simulink library "NullConstraintsBus"  (R2018b)
settings: Solver=VariableStepAuto  StartTime=0.0  StopTime=10.0  RelTol=1e-3
settings Model: Creator=RA24876  LastModifiedBy=RA24876
settings SFSimCC: SimUseLocalCustomCode=off
settings RTWCC: RTWUseLocalCustomCode=off
settings CodeAppCC: StateflowObjectComments=on

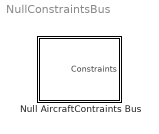
== system NullConstraintsBus ==
  Null AircraftContraints Bus : Subsystem  mask(Null AircraftConstraints Bus){}
      mask help: Creates an AircraftConstraints bus signal with all null values. Assign values to elements with a Bus Assignment block.

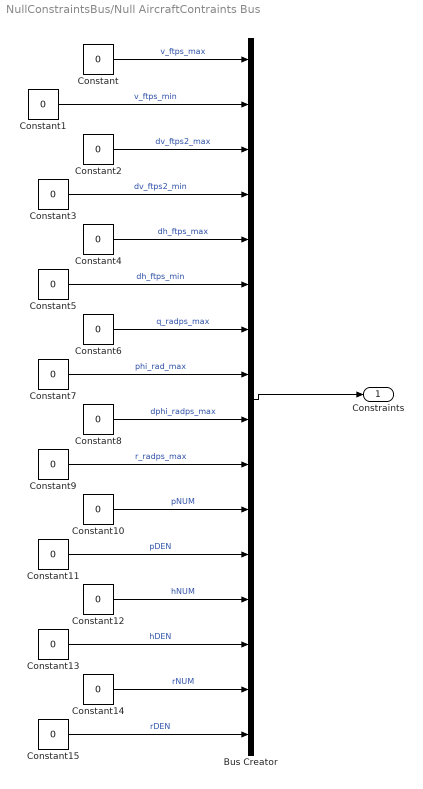
== system NullConstraintsBus/Null AircraftContraints Bus ==
  Bus Creator : BusCreator  Inputs=16  OutDataTypeStr=Bus: AircraftConstraints
      settings: InheritFromInputs=off
  Constant{,1..15} (16 alike) : Constant  Value=0
  Constraints : Outport  OutDataTypeStr=Bus: AircraftConstraints
  wires:
  Bus Creator/1 -> Constraints/1
  Constant/1 -> Bus Creator/1  "v_ftps_max"
  Constant1/1 -> Bus Creator/2  "v_ftps_min"
  Constant2/1 -> Bus Creator/3  "dv_ftps2_max"
  Constant3/1 -> Bus Creator/4  "dv_ftps2_min"
  Constant4/1 -> Bus Creator/5  "dh_ftps_max"
  Constant5/1 -> Bus Creator/6  "dh_ftps_min"
  Constant6/1 -> Bus Creator/7  "q_radps_max"
  Constant7/1 -> Bus Creator/8  "phi_rad_max"
  Constant8/1 -> Bus Creator/9  "dphi_radps_max"
  Constant9/1 -> Bus Creator/10  "r_radps_max"
  Constant10/1 -> Bus Creator/11  "pNUM"
  Constant11/1 -> Bus Creator/12  "pDEN"
  Constant12/1 -> Bus Creator/13  "hNUM"
  Constant13/1 -> Bus Creator/14  "hDEN"
  Constant14/1 -> Bus Creator/15  "rNUM"
  Constant15/1 -> Bus Creator/16  "rDEN"
